simulink model "fro_ut"  (Simulink 8.1)
settings: Solver=FixedStepDiscrete  StartTime=0.0  StopTime=Inf  FixedStep=0.005  RelTol=1e-3
libraries: siltestlib x3, fro x1
settings Model: Creator=xsellart  LastModifiedBy=AT015555
settings DataIOCC: SignalLoggingSaveFormat=Dataset
settings OptimizationCC: ExpressionDepthLimit=128
settings DebuggingCC: FcnCallInpInsideContextMsg=EnableAllAsError
settings GRTTargetCC: CombineOutputUpdateFcns=on  GRTInterface=off

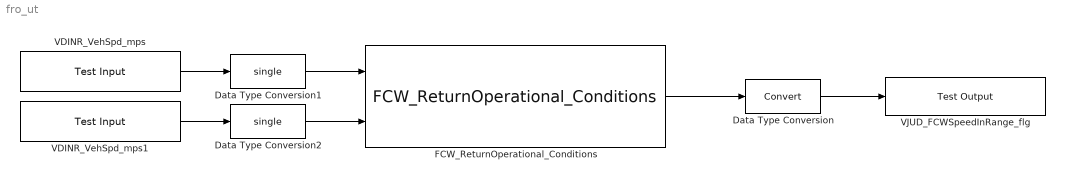
== system fro_ut ==
  Data Type Conversion : DataTypeConversion
  Data Type Conversion1 : DataTypeConversion  OutDataTypeStr=single
  Data Type Conversion2 : DataTypeConversion  OutDataTypeStr=single
  FCW_ReturnOperational_Conditions : fro/FCW_ReturnOperational_Conditions
  VDINR_VehSpd_mps : siltestlib/Test Input  varname=VIFO_FCWTargetVehRelSpeedX_mps  sampletime=0.005
  VDINR_VehSpd_mps1 : siltestlib/Test Input  varname=VIFO_FCWVehClearance_m  sampletime=0.005
  VJUD_FCWSpeedInRange_flg : siltestlib/Test Output  varname=VJUD_FCWReturnOperational_flg  sampletime=-1
  wires:
  VDINR_VehSpd_mps/1 -> Data Type Conversion1/1
  FCW_ReturnOperational_Conditions/1 -> Data Type Conversion/1
  Data Type Conversion/1 -> VJUD_FCWSpeedInRange_flg/1
  Data Type Conversion1/1 -> FCW_ReturnOperational_Conditions/1
  VDINR_VehSpd_mps1/1 -> Data Type Conversion2/1
  Data Type Conversion2/1 -> FCW_ReturnOperational_Conditions/2
